simulink model "rectifier"  (R2015a)
settings: Solver=ode3  StartTime=0.0  StopTime=1  FixedStep=Ts  RelTol=1e-3
values from neighbouring files (symbols this model uses):
  C = 2350e-6    (= 0.00235)    [VOC_param.m]    (also in VOC_param_paper.m = 0.0022; controller_parameters.m = 0.0022; power_control_param.m = 0.002)
  L = 8e-3    (= 0.008)    [VOC_param.m]    (also in VOC_param_paper.m = 0.003; controller_parameters.m = 0.003; current_controller_param.m = 0.005; power_control_param.m = 0.01)
  R = 0.1    [VOC_param.m]    (also in VOC_param_paper.m = 0.05; controller_parameters.m = 0.05; current_controller_param.m; power_control_param.m = 0.3)
  U = 311    [VOC_param.m]    (also in power_control_param.m)
  w = 2*pi*f    (= 314.159265359)    [VOC_param.m]    (also in controller_parameters.m; current_controller_param.m; power_control_param.m)
settings Model: Creator=rblan  LastModifiedBy=rblan

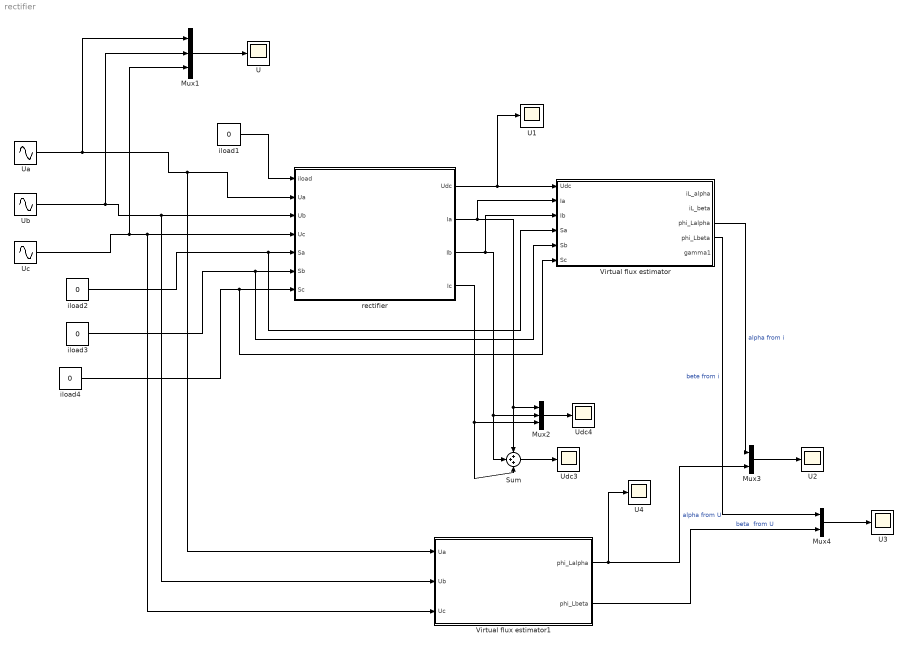
== system rectifier ==
  Mux1 : Mux  Inputs=3
  Mux2 : Mux  Inputs=3
  Mux3 : Mux  Inputs=2
  Mux4 : Mux  Inputs=2
  Sum : Sum  Inputs=+++
  U{,1..4} (5 alike) : Scope
      U settings: ShowLegends=on  YMin=-800  YMax=800  SaveName=Udc_plot
      U1 settings: ShowLegends=on  YMin=-800  YMax=800  SaveName=Udc_plot1
      U2 settings: ShowLegends=on  YMin=-800  YMax=800  SaveName=Udc_plot4
      U3 settings: ShowLegends=on  YMin=-800  YMax=800  SaveName=Udc_plot5
      U4 settings: ShowLegends=on  YMin=-0.25  YMax=2.5  SaveName=Udc_plot6
  Ua : Sin  Amplitude=U  Frequency=w  SampleTime=0
  Ub : Sin  Amplitude=U  Frequency=w  Phase=-2*pi/3  SampleTime=0
  Uc : Sin  Amplitude=U  Frequency=w  Phase=-4*pi/3  SampleTime=0
  Udc3 : Scope
      settings: ShowLegends=on  YMin=-800  YMax=800  SaveName=Udc_plot2
  Udc4 : Scope
      settings: ShowLegends=on  YMin=-800  YMax=800  SaveName=Udc_plot3
  Virtual flux estimator : Subsystem
  Virtual flux estimator1 : Subsystem
  iload{1..4} (4 alike) : Constant  Value=0
  rectifier : Subsystem
  wires:
  Ua/1 -> Virtual flux estimator1/1(Ua), rectifier/2(Ua), Mux1/1
  Ub/1 -> Mux1/2, Virtual flux estimator1/2(Ub), rectifier/3(Ub)
  Uc/1 -> Mux1/3, Virtual flux estimator1/3(Uc), rectifier/4(Uc)
  iload1/1 -> rectifier/1(iload)
  iload2/1 -> Virtual flux estimator/4(Sa), rectifier/5(Sa)
  iload3/1 -> Virtual flux estimator/5(Sb), rectifier/6(Sb)
  iload4/1 -> Virtual flux estimator/6(Sc), rectifier/7(Sc)
  Mux1/1 -> U/1
  Sum/1 -> Udc3/1
  rectifier/4(Ic) -> Mux2/3, Sum/3
  rectifier/2(Ia) -> Virtual flux estimator/2(Ia), Mux2/1, Sum/1
  Mux2/1 -> Udc4/1
  rectifier/3(Ib) -> Virtual flux estimator/3(Ib), Mux2/2, Sum/2
  rectifier/1(Udc) -> U1/1, Virtual flux estimator/1(Udc)
  Virtual flux estimator/3(phi_Lalpha) -> Mux3/1  "alpha from i"
  Virtual flux estimator1/1(phi_Lalpha) -> U4/1, Mux3/2  "alpha from U"
  Mux3/1 -> U2/1
  Virtual flux estimator/4(phi_Lbeta) -> Mux4/1  "bete from i"
  Virtual flux estimator1/2(phi_Lbeta) -> Mux4/2  "beta\t from U"
  Mux4/1 -> U3/1

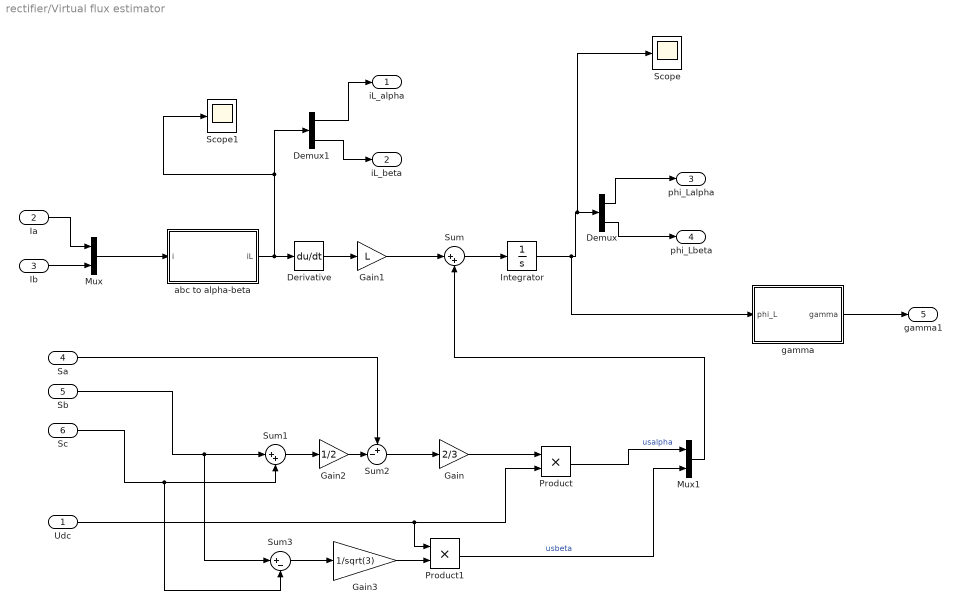
== system rectifier/Virtual flux estimator ==
  Udc : Inport
  Ia : Inport  Port=2
  Ib : Inport  Port=3
  Sa : Inport  Port=4
  Sb : Inport  Port=5
  Sc : Inport  Port=6
  Demux : Demux  Outputs=2
  Demux1 : Demux  Outputs=2
  Derivative : Derivative
  Gain : Gain  Gain=2/3
  Gain1 : Gain  Gain=L
  Gain2 : Gain  Gain=1/2
  Gain3 : Gain  Gain=1/sqrt(3)
  Integrator : Integrator
  Mux : Mux  Inputs=2
  Mux1 : Mux  Inputs=2
  Product : Product
  Product1 : Product
  Scope : Scope
      settings: ShowLegends=on  YMin=-1.5  YMax=1.5
  Scope1 : Scope
      settings: YMin=-450  YMax=450
  Sum : Sum  Inputs=|++
  Sum1 : Sum  Inputs=|++
  Sum2 : Sum  Inputs=+-|
  Sum3 : Sum  Inputs=|+-
  abc to alpha-beta : Subsystem
  gamma : Subsystem
  iL_alpha : Outport
  "iL_beta " : Outport  Port=2
  phi_Lalpha : Outport  Port=3
  phi_Lbeta : Outport  Port=4
  gamma1 : Outport  Port=5
  wires:
  Mux/1 -> abc to alpha-beta/1(i)
  Ia/1 -> Mux/1
  Ib/1 -> Mux/2
  Derivative/1 -> Gain1/1
  Gain1/1 -> Sum/1
  Sb/1 -> Sum3/1, Sum1/1
  Sc/1 -> Sum3/2, Sum1/2
  Sum1/1 -> Gain2/1
  Gain2/1 -> Sum2/2
  Sa/1 -> Sum2/1
  Sum2/1 -> Gain/1
  Gain/1 -> Product/1
  Udc/1 -> Product/2, Product1/1
  Product/1 -> Mux1/1  "usalpha"
  Sum3/1 -> Gain3/1
  Gain3/1 -> Product1/2
  Product1/1 -> Mux1/2  "usbeta"
  abc to alpha-beta/1(iL) -> Demux1/1, Scope1/1, Derivative/1
  Demux1/1 -> iL_alpha/1
  Demux1/2 -> "iL_beta "/1
  Demux/1 -> phi_Lalpha/1
  Demux/2 -> phi_Lbeta/1
  Sum/1 -> Integrator/1
  Integrator/1 -> gamma/1(phi_L), Scope/1, Demux/1
  gamma/1(gamma) -> gamma1/1
  Mux1/1 -> Sum/2

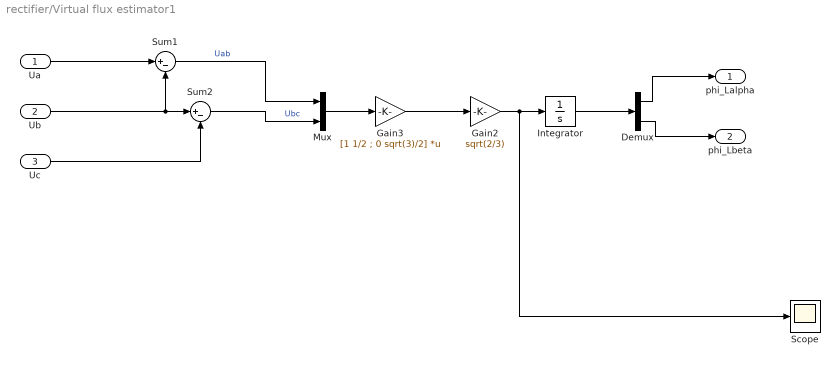
== system rectifier/Virtual flux estimator1 ==
  Ua : Inport
  Ub : Inport  Port=2
  Uc : Inport  Port=3
  Demux : Demux  Outputs=2
  Gain2 : Gain  Gain=sqrt(2/3)
  Gain3 : Gain  Gain=[1 1/2 ; 0 sqrt(3)/2]  Multiplication=Matrix(K*u)
  Integrator : Integrator
  Mux : Mux  Inputs=2
  Scope : Scope
      settings: YMin=-550  YMax=550  SaveName=ScopeData4
  Sum1 : Sum  Inputs=|+-
  Sum2 : Sum  Inputs=|+-
  phi_Lalpha : Outport
  phi_Lbeta : Outport  Port=2
  wires:
  Demux/1 -> phi_Lalpha/1
  Demux/2 -> phi_Lbeta/1
  Integrator/1 -> Demux/1
  Ua/1 -> Sum1/1
  Sum1/1 -> Mux/1  "Uab"
  Ub/1 -> Sum1/2, Sum2/1
  Uc/1 -> Sum2/2
  Sum2/1 -> Mux/2  "Ubc"
  Gain3/1 -> Gain2/1
  Mux/1 -> Gain3/1
  Gain2/1 -> Scope/1, Integrator/1

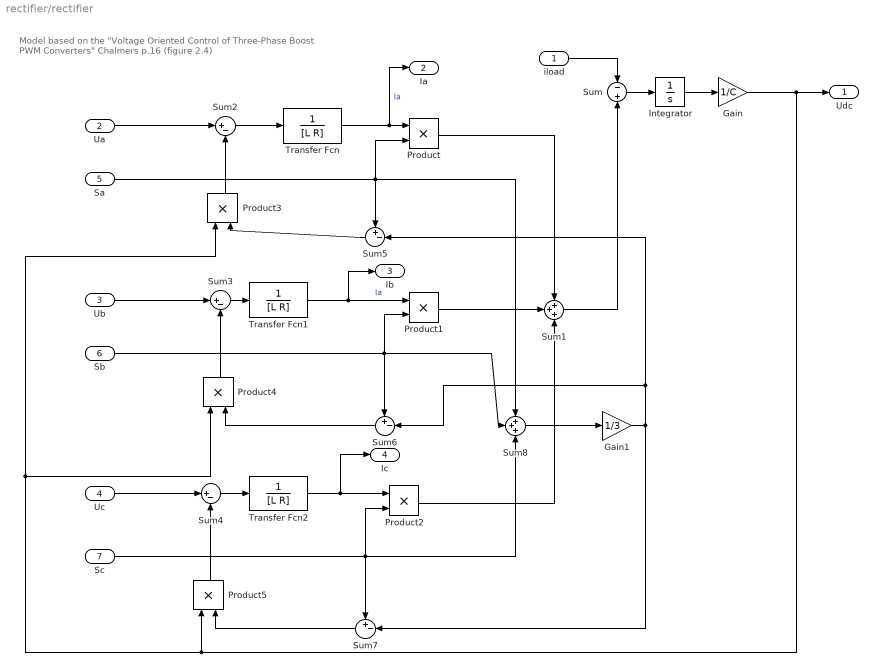
== system rectifier/rectifier ==
  note: Model based on the "Voltage Oriented Control of Three‐Phase
      | Boost PWM Converters" Chalmers p.16 (figure 2.4)
  iload : Inport
  Ua : Inport  Port=2
  Ub : Inport  Port=3
  Uc : Inport  Port=4
  Sa : Inport  Port=5
  Sb : Inport  Port=6
  Sc : Inport  Port=7
  Gain : Gain  Gain=1/C
  Gain1 : Gain  Gain=1/3
  Integrator : Integrator
  Product{,1..5} (6 alike) : Product
  Sum : Sum  Inputs=-|+
  Sum1 : Sum  Inputs=+++
  Sum2 : Sum  Inputs=|+-
  Sum3 : Sum  Inputs=|+-
  Sum4 : Sum  Inputs=|+-
  Sum5 : Sum  Inputs=+-|
  Sum6 : Sum  Inputs=+-|
  Sum7 : Sum  Inputs=+-|
  Sum8 : Sum  Inputs=+++
  Transfer Fcn : TransferFcn  Denominator=[L R]
  Transfer Fcn1 : TransferFcn  Denominator=[L R]
  Transfer Fcn2 : TransferFcn  Denominator=[L R]
  Udc : Outport
  Ia : Outport  Port=2
  Ib : Outport  Port=3
  Ic : Outport  Port=4
  wires:
  Gain/1 -> Product5/1, Product3/1, Product4/1, Udc/1
  Integrator/1 -> Gain/1
  iload/1 -> Sum/1
  Sum1/1 -> Sum/2
  Product/1 -> Sum1/1
  Product1/1 -> Sum1/2
  Product2/1 -> Sum1/3
  Transfer Fcn/1 -> Ia/1, Product/1  "Ia"
  Transfer Fcn1/1 -> Ib/1, Product1/1  "Ia"
  Transfer Fcn2/1 -> Ic/1, Product2/1
  Sum2/1 -> Transfer Fcn/1
  Ua/1 -> Sum2/1
  Product3/1 -> Sum2/2
  Sum3/1 -> Transfer Fcn1/1
  Sum4/1 -> Transfer Fcn2/1
  Ub/1 -> Sum3/1
  Uc/1 -> Sum4/1
  Sa/1 -> Sum8/1, Product/2, Sum5/1
  Sb/1 -> Sum6/1, Sum8/2, Product1/2
  Sc/1 -> Sum8/3, Sum7/1, Product2/2
  Product4/1 -> Sum3/2
  Product5/1 -> Sum4/2
  Sum5/1 -> Product3/2
  Sum6/1 -> Product4/2
  Sum7/1 -> Product5/2
  Sum/1 -> Integrator/1
  Sum8/1 -> Gain1/1
  Gain1/1 -> Sum6/2, Sum5/2, Sum7/2

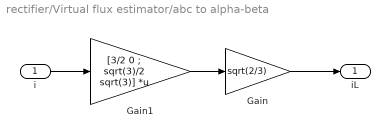
== system rectifier/Virtual flux estimator/abc to alpha-beta ==
  i : Inport
  Gain : Gain  Gain=sqrt(2/3)
  Gain1 : Gain  Gain=[3/2 0 ; sqrt(3)/2 sqrt(3)]  Multiplication=Matrix(K*u)
  iL : Outport
  wires:
  Gain1/1 -> Gain/1
  i/1 -> Gain1/1
  Gain/1 -> iL/1

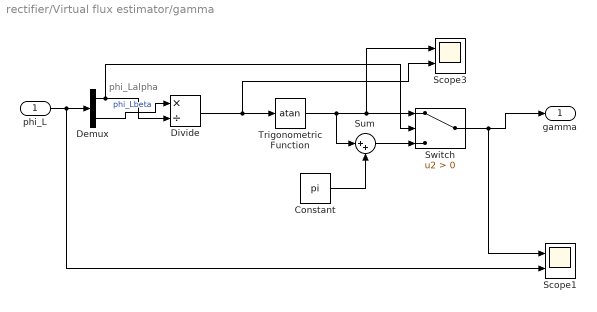
== system rectifier/Virtual flux estimator/gamma ==
  note: phi_Lalpha
  phi_L : Inport
  Constant : Constant  Value=pi
  Demux : Demux  Outputs=2
  Divide : Product  Inputs=*/
  Scope1 : Scope  NumInputPorts=2
      settings: ShowLegends=on  YMin=-2~-1.25  YMax=5~2  SaveName=ScopeData3
  Scope3 : Scope  NumInputPorts=2
      settings: YMin=-1.75~-500  YMax=1.75~300  SaveName=ScopeData2
  Sum : Sum  Inputs=|++
  Switch : Switch  Criteria=u2 > Threshold
  Trigonometric Function : Trigonometry  Operator=atan
  gamma : Outport
  wires:
  phi_L/1 -> Scope1/2, Demux/1
  Demux/1 -> Divide/2, Switch/2
  Demux/2 -> Divide/1  "phi_Lbeta"
  Constant/1 -> Sum/2
  Divide/1 -> Scope3/2, Trigonometric Function/1
  Trigonometric Function/1 -> Sum/1, Scope3/1, Switch/1
  Sum/1 -> Switch/3
  Switch/1 -> Scope1/1, gamma/1
